simulink model "lab06z5_sch"  (R2022b)
settings: Solver=ode23t  StartTime=0.0  StopTime=12  RelTol=1e-6  EnableMultiTasking=on
settings Model: Creator=Jacek  LastModifiedBy=Robert
settings SolverCC: AlgebraicLoopSolver=TrustRegion
settings DataIOCC: LimitDataPoints=on  SaveFormat=Array  SignalLoggingSaveFormat=ModelDataLogs  ReturnWorkspaceOutputs=off  SignalLoggingName=sigsOut
settings OptimizationCC: BooleanDataType=off  InitFltsAndDblsToZero=on  LifeSpan=inf
settings DebuggingCC: SaveWithParameterizedLinksMsg=none  UnderspecifiedInitializationDetection=Classic  MergeDetectMultiDrivingBlocksExec=none  SignalResolutionControl=TryResolveAllWithWarning  MultiTaskDSMMsg=warning  MultiTaskCondExecSysMsg=none  FcnCallInpInsideContextMsg=warning  UnconnectedInputMsg=warning  UnconnectedOutputMsg=warning  UnconnectedLineMsg=warning  SFUnexpectedBacktrackingDiag=warning  SFNoUnconditionalDefaultTransitionDiag=warning  SFExecutionAtInitializationDiag=none  SFMachineParentedDataDiag=warning  ArithmeticOperatorsInVariantConditions=warning
settings HardwareCC: ProdBitPerPointer=32  ProdBitPerSizeT=32  ProdBitPerPtrDiffT=32  ProdLargestAtomicFloat=None  ProdIntDivRoundTo=Undefined  ProdEndianess=Unspecified  ProdWordSize=32  ProdHWDeviceType=32-bit Generic  TargetUnknown=on
settings ModelReferenceCC: EnableRefExpFcnMdlSchedulingChecks=on  PropagateSignalLabelsOutOfModel=off
settings SFSimCC: SimUseLocalCustomCode=off  CustomCodeUndefinedFunction=UseInterfaceOnly
settings RTWCC: RTWUseLocalCustomCode=off
settings CodeAppCC: StateflowObjectComments=on
settings GRTTargetCC: TargetFcnLib=ansi_tfl_tmw.mat  TargetLangStandard=C89/C90 (ANSI)  CombineOutputUpdateFcns=off  GRTInterface=on
settings ConfigComp: CovMetricSettings=dw  CovSaveCumulativeToWorkspaceVar=on  CovSaveSingleToWorkspaceVar=on  CovExternalEMLEnable=off

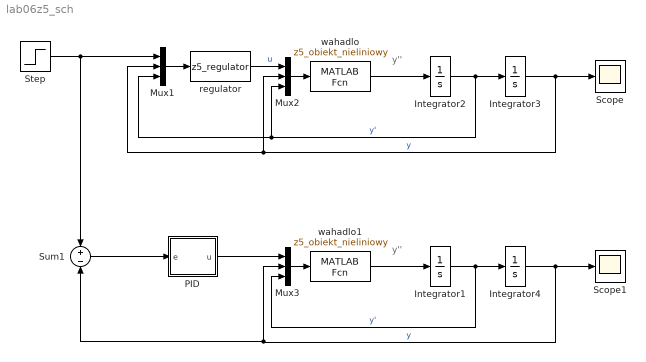
== system lab06z5_sch ==
  note: y''
  note: y''
  Integrator{1..4} (4 alike) : Integrator
  Mux1 : Mux  Inputs=3
  Mux2 : Mux  Inputs=3
  Mux3 : Mux  Inputs=3
  PID : Subsystem
  Scope : Scope
  Scope1 : Scope
  Step : Step  Time=0  After=6.28  SampleTime=0
  Sum1 : Sum  Inputs=+|-
  regulator : MATLABFcn  MATLABFcn=z5_regulator
  wahadlo : MATLABFcn  MATLABFcn=z5_obiekt_nieliniowy
  wahadlo1 : MATLABFcn  MATLABFcn=z5_obiekt_nieliniowy  OutputDimensions=1
  wires:
  wahadlo/1 -> Integrator2/1
  Integrator2/1 -> Mux2/3, Mux1/3, Integrator3/1  "y'"
  Integrator3/1 -> Scope/1, Mux2/2, Mux1/2  "y"
  Mux2/1 -> wahadlo/1
  Mux1/1 -> regulator/1
  regulator/1 -> Mux2/1  "u"
  Step/1 -> Sum1/1, Mux1/1
  Mux3/1 -> wahadlo1/1
  wahadlo1/1 -> Integrator1/1
  Integrator1/1 -> Mux3/3, Integrator4/1  "y'"
  Integrator4/1 -> Scope1/1, Sum1/2, Mux3/2  "y"
  Sum1/1 -> PID/1(e)
  PID/1(u) -> Mux3/1

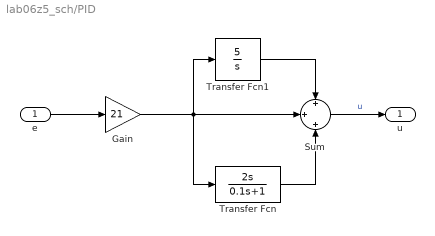
== system lab06z5_sch/PID ==
  e : Inport
  Gain : Gain  Gain=21
  Sum : Sum  Inputs=+|+|+
  Transfer Fcn : TransferFcn  Numerator=[2 0]  Denominator=[0.1 1]
  Transfer Fcn1 : TransferFcn  Numerator=[5]  Denominator=[1 0]
  u : Outport  VectorParamsAs1DForOutWhenUnconnected=off
  wires:
  Transfer Fcn1/1 -> Sum/1
  e/1 -> Gain/1
  Sum/1 -> u/1  "u"
  Transfer Fcn/1 -> Sum/3
  Gain/1 -> Sum/2, Transfer Fcn/1, Transfer Fcn1/1
